simulink model "lab3"  (R2021a)
settings: Solver=FixedStepAuto  StartTime=0.0  StopTime=10.0  FixedStep=1e-3  RelTol=1e-3
settings Model: Creator=Beshary  LastModifiedBy=Beshary

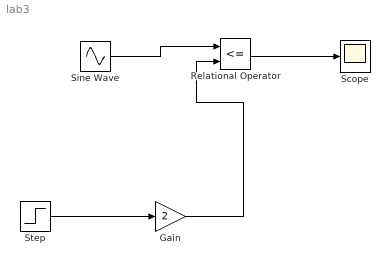
== system lab3 ==
  Gain : Gain  Gain=2
  Relational Operator : RelationalOperator  Operator=<=  OutDataTypeStr=boolean  RndMeth=Simplest
  Scope : Scope
  Sine Wave : Sin  Frequency=2*pi  SampleTime=0
  Step : Step  SampleTime=2
  wires:
  Sine Wave/1 -> Relational Operator/1
  Relational Operator/1 -> Scope/1
  Step/1 -> Gain/1
  Gain/1 -> Relational Operator/2
